simulink model "JAKDZIALAMUX"  (R2020b)
settings: Solver=VariableStepAuto  StartTime=0.0  StopTime=10.0  RelTol=1e-3
settings Model: Creator=Adam  LastModifiedBy=Adam

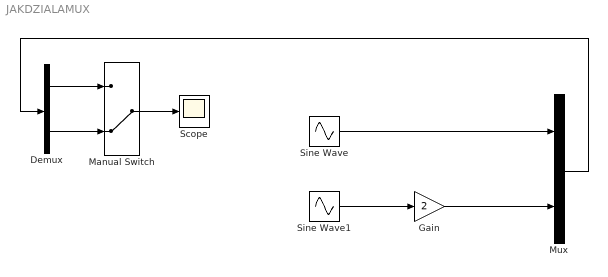
== system JAKDZIALAMUX ==
  Demux : Demux  Outputs=2
  Gain : Gain  Gain=2
  Manual Switch : ManualSwitch  CurrentSetting=0
  Mux : Mux  Inputs=2
  Scope : Scope
  Sine Wave : Sin  SampleTime=0
  Sine Wave1 : Sin  SampleTime=0
  wires:
  Mux/1 -> Demux/1
  Demux/1 -> Manual Switch/1
  Demux/2 -> Manual Switch/2
  Manual Switch/1 -> Scope/1
  Sine Wave1/1 -> Gain/1
  Sine Wave/1 -> Mux/1
  Gain/1 -> Mux/2
